simulink model "FieldOrientedController_MIL"  (R2020a)
settings: configuration reference "Sim" (kept outside this file)
undefined symbols (not defined in the file): commandTypeEnum, encoder, paramAdcTransducerVoltAtZeroAmpere, pmsm
libraries: SignalEditorBlockLib x1
settings Model: DataDictionary=focRCP_Data.sldd  EnableAccessToBaseWorkspace=off  PauseTimes=0  NumberOfSteps=10  OrderedModelArguments=off  Creator=promero  LastModifiedBy=manuel.fedou
settings ConfigSetRef: SourceName=Sim

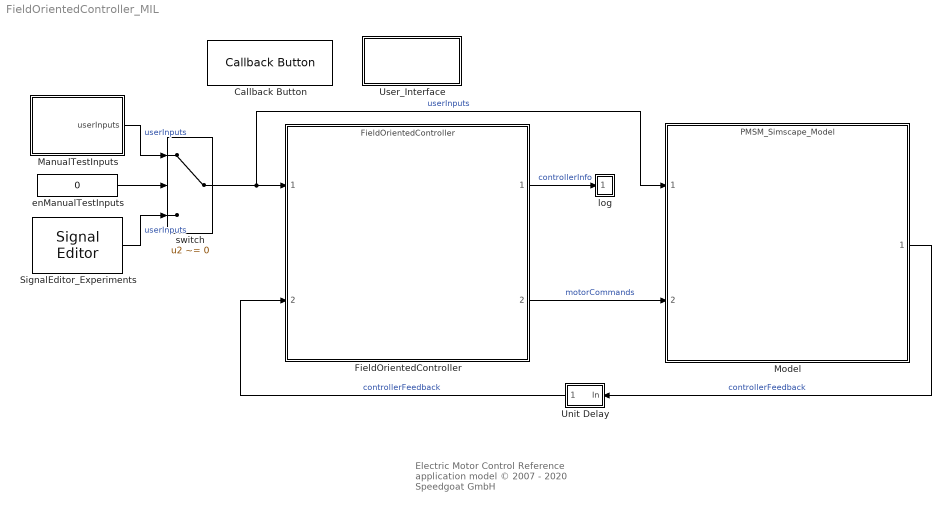
== system FieldOrientedController_MIL ==
  note: Electric Motor Control
      | Reference application model
      | © 2007 - 2020 Speedgoat GmbH
  Callback Button : CallbackButton  ButtonText=Switch Electric Motor Control Kit
      settings: ClickFcn=|
      | SelectMotorKit
      | set_param(gcs,'SimulationCommand','Update')
  FieldOrientedController : ModelReference  ModelNameDialog=FieldOrientedController  SimulationMode=Normal  ModelReferenceVersion=1.608
      mask Display: image('focVelocityEncoderHwSwCMask.png');
  ManualTestInputs : Subsystem  Description=""  VariantControl=TestInputChoice == 2
      settings: RTWSystemCode=Nonreusable function
  Model : ModelReference  ModelNameDialog=PMSM_Simscape_Model.slx  SimulationMode=Normal  ModelReferenceVersion=1.376
      mask Display: image('focVelocityEncoderMotorAndLoadAvgVoltageMask.png'); % Use "Edit Image" on toolstrip to change.
  SignalEditor_Experiments : SignalEditorBlockLib/Signal Editor  FileName=PMSM_Experiments.mat  ActiveScenario=ClosedLoop_CoastdownTest  ActiveSignal=userInputs  IsBus=on  OutputBusObjectStr=Bus: userInputs  SampleTime=-1  Interpolate=off  ZeroCross=off  OutputAfterFinalValue=Holding final value  Unit=inherit  PreserveSignalName=on
  Unit Delay : Subsystem
  User_Interface : Subsystem
  enManualTestInputs : Constant  Value=0  OutDataTypeStr=boolean
  log : Subsystem
  switch : Switch  Criteria=u2 ~= 0
  wires:
  Model/1 -> Unit Delay/1(In)  "controllerFeedback"
  switch/1 -> Model/1, FieldOrientedController/1  "userInputs"
  SignalEditor_Experiments/1 -> switch/3  "userInputs"
  ManualTestInputs/1(userInputs) -> switch/1  "userInputs"
  enManualTestInputs/1 -> switch/2
  Unit Delay/1(Out) -> FieldOrientedController/2  "controllerFeedback"
  FieldOrientedController/2 -> Model/2  "motorCommands"
  FieldOrientedController/1 -> log/1(In)  "controllerInfo"

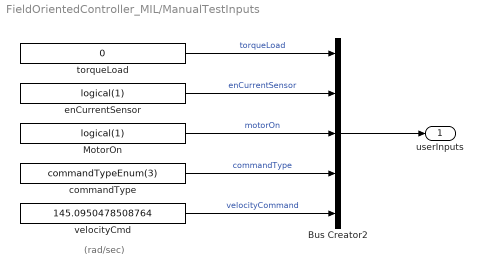
== system FieldOrientedController_MIL/ManualTestInputs ==
  note: (rad/sec)
  Bus Creator2 : BusCreator  Inputs=5  OutDataTypeStr=Bus: userInputs  NonVirtualBus=on
      settings: InheritFromInputs=off
  MotorOn : Constant  Value=logical(1)  OutDataTypeStr=boolean  SampleTime=-1
  commandType : Constant  Value=commandTypeEnum(3)  SampleTime=-1
  enCurrentSensor : Constant  Value=logical(1)  OutDataTypeStr=boolean  SampleTime=-1
  torqueLoad : Constant  Value=0  OutDataTypeStr=double  SampleTime=-1
  velocityCmd : Constant  Value=145.0950478508764  OutDataTypeStr=single  SampleTime=-1
  userInputs : Outport  VectorParamsAs1DForOutWhenUnconnected=off
  wires:
  MotorOn/1 -> Bus Creator2/3  "motorOn"
  commandType/1 -> Bus Creator2/4  "commandType"
  torqueLoad/1 -> Bus Creator2/1  "torqueLoad"
  enCurrentSensor/1 -> Bus Creator2/2  "enCurrentSensor"
  Bus Creator2/1 -> userInputs/1
  velocityCmd/1 -> Bus Creator2/5  "velocityCommand"

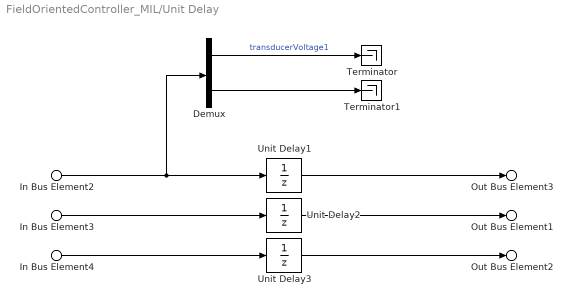
== system FieldOrientedController_MIL/Unit Delay ==
  In Bus Element2 : Inport  PortName=In  Element=transducerVoltage
  In Bus Element3 : Inport  PortName=In  Element=encoderIndexFound
  In Bus Element4 : Inport  PortName=In  Element=encoderCount
  Demux : Demux  Outputs=2
  Terminator : Terminator
  Terminator1 : Terminator
  Unit Delay1 : UnitDelay  InitialCondition=paramAdcTransducerVoltAtZeroAmpere  SampleTime=-1  HasFrameUpgradeWarning=on
  Unit Delay2 : UnitDelay  InitialCondition=1  SampleTime=-1  HasFrameUpgradeWarning=on
  Unit Delay3 : UnitDelay  InitialCondition=uint16((pmsm.RotorPositionInit-encoder.RotorPositionAtIndex)*encoder.CountPerRevolution/(2*pi))  SampleTime=-1  HasFrameUpgradeWarning=on
  Out Bus Element3 : Outport  PortName=Out  Element=transducerVoltage
  Out Bus Element1 : Outport  PortName=Out  Element=encoderIndexFound
  Out Bus Element2 : Outport  PortName=Out  Element=encoderCount
  wires:
  In Bus Element2/1 -> Demux/1, Unit Delay1/1
  In Bus Element3/1 -> Unit Delay2/1
  In Bus Element4/1 -> Unit Delay3/1
  Unit Delay1/1 -> Out Bus Element3/1
  Unit Delay2/1 -> Out Bus Element1/1
  Unit Delay3/1 -> Out Bus Element2/1
  Demux/1 -> Terminator/1  "transducerVoltage1"
  Demux/2 -> Terminator1/1

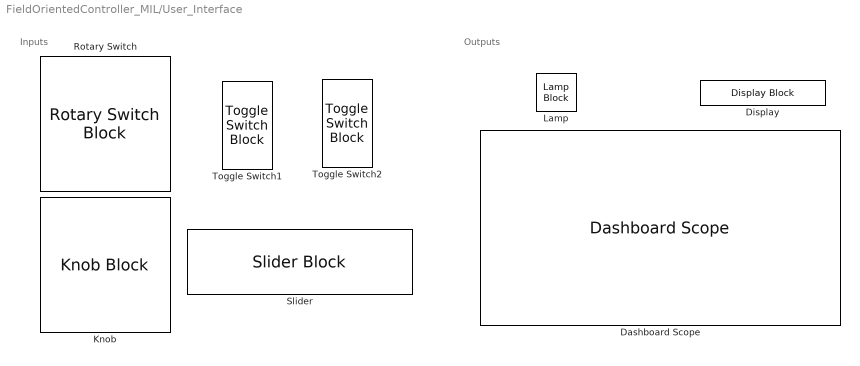
== system FieldOrientedController_MIL/User_Interface ==
  note: Inputs
  note: Outputs
  Dashboard Scope : DashboardScope  TimeSpan=10  Ymin=-250  Ymax=250  ScaleAtStop=off
  Display : DisplayBlock  LabelPosition=Hide  Format=short  Transparency=1
  Knob : KnobBlock  ScaleMin=-250  ScaleMax=250  TickInterval=50
  Lamp : LampBlock
  Rotary Switch : RotarySwitchBlock  UseEnumeratedDataType=on  EnumeratedDataType=commandTypeEnum
      settings: Values={{'Error', 'OpenLoop', 'CalibrateEncoder', 'ClosedLoop'}, [0 1 2 3]}
  Slider : SliderBlock  ScaleMin=-1  ScaleMax=1  TickInterval=0.25
  Toggle Switch1 : ToggleSwitchBlock
      settings: Values={{'Off', 'On'}, [0 1]}
  Toggle Switch2 : ToggleSwitchBlock
      settings: Values={{'Off', 'On'}, [0 1]}

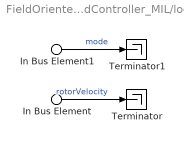
== system FieldOrientedController_MIL/log ==
  In Bus Element1 : Inport  PortName=In  Element=mode
  In Bus Element : Inport  PortName=In  Element=rotorVelocity
  Terminator : Terminator
  Terminator1 : Terminator
  wires:
  In Bus Element/1 -> Terminator/1  "rotorVelocity"
  In Bus Element1/1 -> Terminator1/1  "mode"
